simulink model "lqr_controls"  (R2018a)
settings: Solver=ode45  StartTime=0.0  StopTime=30  RelTol=1e-3
settings Model: Creator=HARSH  LastModifiedBy=HARSH

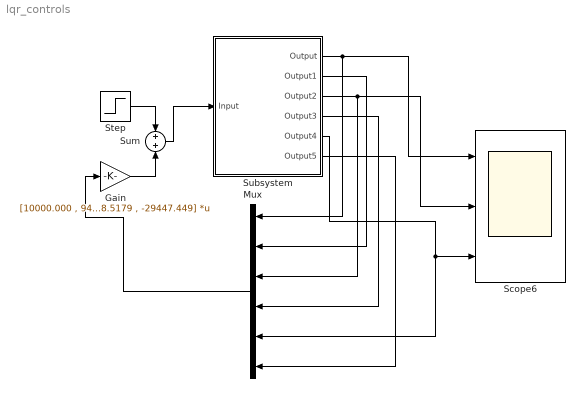
== system lqr_controls ==
  Gain : Gain  Gain="[10000.000 , 9495.4117 ,  21169.4517 , -32255.5023 , 11278.5179 , -29447.449]"  Multiplication=Matrix(K*u)
  Mux : Mux  Inputs=6
  Scope6 : Scope  NumInputPorts=3
  Step : Step  After=500  SampleTime=0  VectorParams1D=off
  Subsystem : Subsystem
  Sum : Sum  Inputs=2
  wires:
  Subsystem/1(Output) -> Scope6/1, Mux/1
  Subsystem/2(Output1) -> Mux/2
  Subsystem/3(Output2) -> Mux/3, Scope6/2
  Subsystem/4(Output3) -> Mux/4
  Subsystem/5(Output4) -> Mux/5, Scope6/3
  Subsystem/6(Output5) -> Mux/6
  Mux/1 -> Gain/1
  Gain/1 -> Sum/2
  Sum/1 -> Subsystem/1(Input)
  Step/1 -> Sum/1

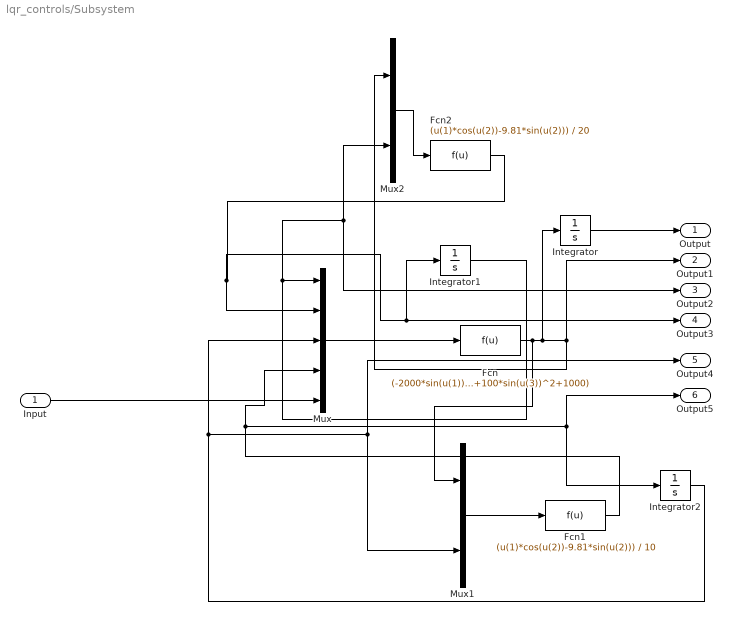
== system lqr_controls/Subsystem ==
  Input : Inport
  Fcn : Fcn  Expr=(-2000*sin(u(1))*u(2)^2 + 1000*sin(u(3))*u(4)^2-u(5)+981*cos(u(1))*sin(u(1))+981*cos(u(3))*sin(u(3)))/(100*sin(u(1))^2+100*sin(u(3))^2+1000)
  Fcn1 : Fcn  Expr=(u(1)*cos(u(2))-9.81*sin(u(2))) / 10
  Fcn2 : Fcn  Expr=(u(1)*cos(u(2))-9.81*sin(u(2))) / 20
  Integrator : Integrator  InitialCondition=1
  Integrator1 : Integrator  InitialCondition=.2
  Integrator2 : Integrator  InitialCondition=.2
  Mux : Mux  Inputs=5
  Mux1 : Mux  Inputs=2
  Mux2 : Mux  Inputs=2
  Output : Outport
  Output1 : Outport  Port=2
  Output2 : Outport  Port=3
  Output3 : Outport  Port=4
  Output4 : Outport  Port=5
  Output5 : Outport  Port=6
  wires:
  Fcn/1 -> Mux1/1, Integrator/1, Output1/1, Mux2/1
  Input/1 -> Mux/5
  Integrator/1 -> Output/1
  Integrator2/1 -> Mux/3, Output4/1, Mux1/2
  Mux1/1 -> Fcn1/1
  Integrator1/1 -> Output2/1, Mux2/2, Mux/1
  Fcn1/1 -> Mux/4, Output5/1, Integrator2/1
  Mux2/1 -> Fcn2/1
  Fcn2/1 -> Mux/2, Output3/1, Integrator1/1
  Mux/1 -> Fcn/1
